simulink model "ep_p_4_29"  (R2023b)
settings: Solver=VariableStepAuto  StartTime=0.0  StopTime=10.0  MaxStep=0.01  RelTol=1e-3  AbsTol=1e-6
settings Model: Creator=86186  LastModifiedBy=86186

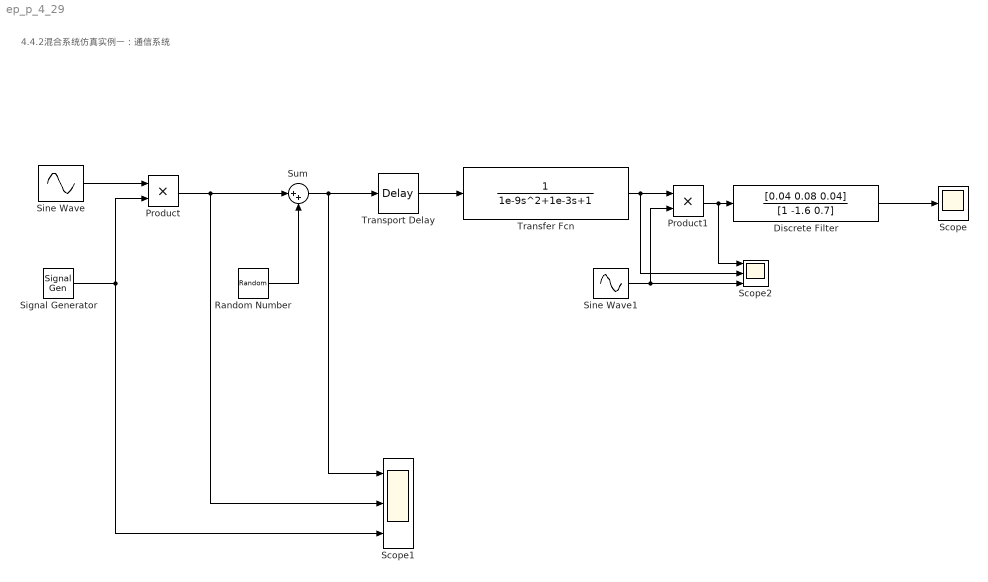
== system ep_p_4_29 ==
  note: 4.4.2混合系统仿真实例一：通信系统
  Discrete Filter : DiscreteFilter  Numerator=[0.04 0.08 0.04]  Denominator=[1 -1.6 0.7]
  Product : Product
  Product1 : Product
  Random Number : RandomNumber  Variance=0.01  SampleTime=0.1
  Scope : Scope
  Scope1 : Scope  NumInputPorts=3
  Scope2 : Scope  NumInputPorts=3
  Signal Generator : SignalGenerator  WaveForm=sawtooth  Frequency=2*pi  Units=rad/sec
  Sine Wave : Sin  Frequency=100  SampleTime=0
  Sine Wave1 : Sin  Frequency=100  SampleTime=0.005
  Sum : Sum  Inputs=|++
  Transfer Fcn : TransferFcn  Denominator=[1e-9 1e-3 1]
  Transport Delay : TransportDelay
  wires:
  Sine Wave/1 -> Product/1
  Signal Generator/1 -> Scope1/3, Product/2
  Random Number/1 -> Sum/2
  Sum/1 -> Scope1/1, Transport Delay/1
  Transport Delay/1 -> Transfer Fcn/1
  Transfer Fcn/1 -> Product1/1, Scope2/2
  Sine Wave1/1 -> Scope2/3, Product1/2
  Product1/1 -> Scope2/1, Discrete Filter/1
  Product/1 -> Scope1/2, Sum/1
  Discrete Filter/1 -> Scope/1
